simulink model "axi_qpsk_rx_dec"  (R2017b)
settings: Solver=VariableStepAuto  StartTime=0.0  StopTime=10.0  RelTol=1e-3
PreLoadFcn:
  | design_filters_rx;      % run script to generate filter designs.
  | 
  | Rb = 1000;   % 1kbit / s
  | 
  | Rsym = Rb/2;   % 2 bits per symbol
  | 
  | Rsymbol = Rb/2;
  | 
  | OSR = 32;
  | 
  | f_error = 120;
  | 
  | fc = 100e3;
InitFcn:
  | fs_in=25.6e6;
values from neighbouring files (symbols this model uses):
  R_CIC = 3200    [design_filters_rx.m]
  R_CICcomp = 2    [design_filters_rx.m]
  R_HB = 2    [design_filters_rx.m]
  R_RRC = 4    [design_filters_rx.m]
undefined symbols (not defined in the file or in its folder): AXI4, designMultirateFIR, Lite
libraries: xbsIndex_r4 x70, dspmlti4 x12, dsparch4 x2, dspsrcs4 x2, commrandsrc2 x1, commdigbbndpm3 x1
settings Model: SimulationMode=accelerator  Creator=jgoldsmi  LastModifiedBy=josh

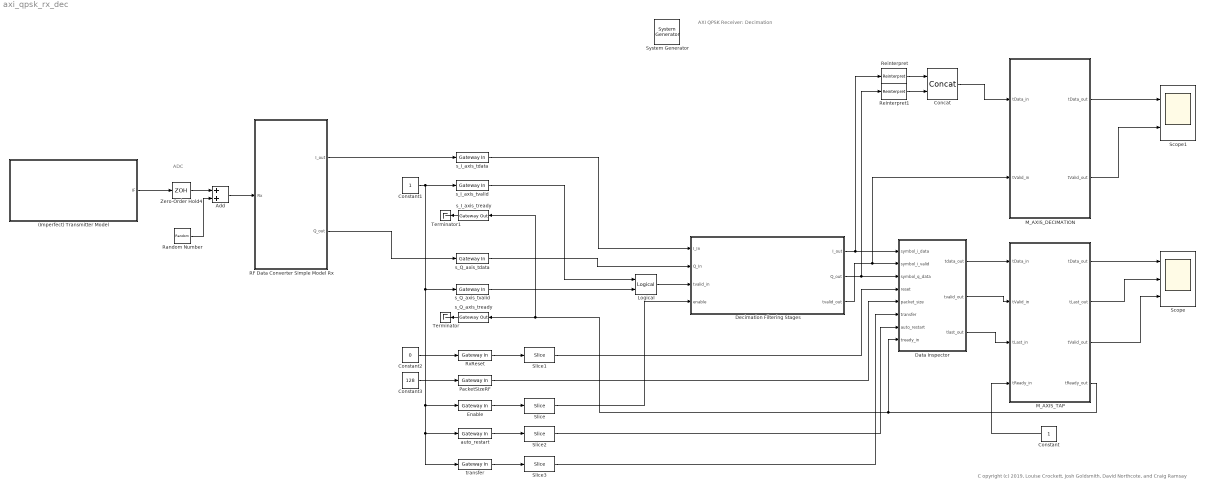
== system axi_qpsk_rx_dec ==
  note: ADC
  note: C opyright (c) 2019, Louise Crockett, Josh Goldsmith, David Northcote, and Craig Ramsay
  note: AXI QPSK Receiver:
      | Decimation
  " System Generator" : xbsIndex_r4/ System Generator  Tag=genX  xilinxfamily=zynquplusRFSOC  part=xczu28dr  speed=-2-e  package=ffvg1517  synthesis_tool=Vivado  clock_wrapper=Clock Enables  directory=../iprepo/zcu111/rx/rx_decimation  proj_type=Vivado  Synth_file=Vivado Synthesis Defaults  Impl_file=Vivado Implementation Defaults  testbench=off  simulink_period=1/fs_in  sysclk_period=(1/fs_in)/1e-9  dcm_input_clock_period=10  incr_netlist=off  trim_vbits=Everywhere in SubSystem  dbl_ovrd=According to Block Masks  core_generation=According to Block Masks  run_coregen=off  deprecated_control=off  eval_field=0  block_type=sysgen
  (Imperfect) Transmitter Model : Subsystem  mask(Model of a QPSK Transmitter with Timing and Frequency Offsets){T_error=5, F_error=f_error, fc=fc}
      mask prompts: T_error "Timing Error (ppm)"; F_error "Frequency Error (Hz)"; fc "IF Carrier Frequency (Hz)"
      mask help:
      | Enter the timing and frequency offsets that apply to the received signal.
      |
      | Both of these can be negative or positive values. Negative means that the timing / frequency of the transmitter is lower than expected.
      mask init:
      | T_Offset = 1+(T_error/1e6);
      | F_Offset = F_error;
  Add : Sum
  Concat : xbsIndex_r4/Concat  num_inputs=2  dbl_ovrd=off  block_type=concat
  Constant : Constant  OutDataTypeStr=boolean  SampleTime=1/fs_in
  Constant1 : Constant  OutDataTypeStr=boolean  SampleTime=-1
  Constant2 : Constant  Value=0  OutDataTypeStr=boolean  SampleTime=-1
  Constant3 : Constant  Value=128  OutDataTypeStr=uint32  SampleTime=-1
  Data Inspector : Subsystem
  Decimation Filtering Stages : Subsystem
  Enable : xbsIndex_r4/Gateway In  gui_display_data_type=Fixed-point  arith_type=Unsigned  n_bits=32  bin_pt=0  preci_type=Single  exp_width=8  frac_width=24  rows=1  columns=1  quantization="Round  (unbiased: +/- Inf)"  overflow=Saturate  period=1/fs_in  UseAsADC=off  ADCChannel='1'  interface=AXI4-Lite  automatic_assignment=off  address_offset=8  intf_name=''  intf_description=''  default_value=0  timing_constraint=None  locs_specified=off  LOCs={}  io_standard={}  inherit_from_input=off  hdl_port=on  dbl_ovrd=off  block_type=gatewayin
  Logical : xbsIndex_r4/Logical  logical_function=AND  inputs=2  en=off  latency=1  precision=Full  arith_type=Unsigned  n_bits=16  bin_pt=0  align_bp=on  dbl_ovrd=off  block_type=logical
  M_AXIS_DECIMATION : Subsystem
  M_AXIS_TAP : Subsystem
  PacketSizeRF : xbsIndex_r4/Gateway In  gui_display_data_type=Fixed-point  arith_type=Unsigned  n_bits=32  bin_pt=0  preci_type=Single  exp_width=8  frac_width=24  rows=1  columns=1  quantization=Truncate  overflow=Wrap  period=1/fs_in  UseAsADC=off  ADCChannel='1'  interface=AXI4-Lite  automatic_assignment=off  address_offset=4  intf_name=''  intf_description=''  default_value=0  timing_constraint=None  locs_specified=off  LOCs={}  io_standard={}  inherit_from_input=off  hdl_port=on  dbl_ovrd=off  block_type=gatewayin
  RF Data Converter Simple Model Rx : Subsystem
  Random Number : RandomNumber  Variance=0.05  SampleTime=1/(0.5*R_RRC*R_HB*R_CICcomp*R_CIC*8*Rb)
  Reinterpret : xbsIndex_r4/Reinterpret  force_arith_type=on  arith_type=Unsigned  force_bin_pt=on  bin_pt=0  block_type=reinterpret
  Reinterpret1 : xbsIndex_r4/Reinterpret  force_arith_type=on  arith_type=Unsigned  force_bin_pt=on  bin_pt=0  block_type=reinterpret
  RxReset : xbsIndex_r4/Gateway In  gui_display_data_type=Fixed-point  arith_type=Unsigned  n_bits=32  bin_pt=0  preci_type=Single  exp_width=8  frac_width=24  rows=1  columns=1  quantization="Round  (unbiased: +/- Inf)"  overflow=Saturate  period=1/fs_in  UseAsADC=off  ADCChannel='1'  interface=AXI4-Lite  automatic_assignment=off  address_offset=0  intf_name=''  intf_description=''  default_value=0  timing_constraint=None  locs_specified=off  LOCs={}  io_standard={}  inherit_from_input=off  hdl_port=on  dbl_ovrd=off  block_type=gatewayin
  Scope : Scope  NumInputPorts=3
  Scope1 : Scope  NumInputPorts=2
  Slice{,1..3} (4 alike) : xbsIndex_r4/Slice  nbits=1  boolean_output=on  mode=Two Bit Locations  bit1=0  base1=LSB of Input  bit0=0  base0=LSB of Input  dbl_ovrd=off  block_type=slice
  Terminator : Terminator
  Terminator1 : Terminator
  Zero-Order Hold4 : ZeroOrderHold  SampleTime=1/(0.5*R_RRC*R_HB*R_CICcomp*R_CIC*8*Rb)
  auto_restart : xbsIndex_r4/Gateway In  gui_display_data_type=Fixed-point  arith_type=Unsigned  n_bits=32  bin_pt=0  preci_type=Single  exp_width=8  frac_width=24  rows=1  columns=1  quantization="Round  (unbiased: +/- Inf)"  overflow=Saturate  period=1/fs_in  UseAsADC=off  ADCChannel='1'  interface=AXI4-Lite  automatic_assignment=off  address_offset=12  intf_name=''  intf_description=''  default_value=0  timing_constraint=None  locs_specified=off  LOCs={}  io_standard={}  inherit_from_input=off  hdl_port=on  dbl_ovrd=off  block_type=gatewayin
  s_I_axis_tdata : xbsIndex_r4/Gateway In  gui_display_data_type=Fixed-point  arith_type="Signed  (2's comp)"  n_bits=16  bin_pt=14  preci_type=Single  exp_width=8  frac_width=24  rows=1  columns=1  quantization="Round  (unbiased: +/- Inf)"  overflow=Saturate  period=1/fs_in  UseAsADC=off  ADCChannel='1'  interface=None  automatic_assignment=on  address_offset=hex2dec('00')  intf_name=''  intf_description=''  default_value=0  timing_constraint=None  locs_specified=off  LOCs={}  io_standard={}  inherit_from_input=off  hdl_port=on  dbl_ovrd=off  block_type=gatewayin
  s_I_axis_tready : xbsIndex_r4/Gateway Out  inherit_from_input=off  hdl_port=on  rows=1  columns=1  UseAsDAC=off  DACChannel='1'  interface=None  automatic_assignment=on  address_offset=hex2dec('00')  intf_name=''  intf_description=''  timing_constraint=None  locs_specified=off  LOCs={}  io_standard={}  block_type=gatewayout
  s_I_axis_tvalid : xbsIndex_r4/Gateway In  gui_display_data_type=Boolean  arith_type=Boolean  n_bits=32  bin_pt=0  preci_type=Single  exp_width=8  frac_width=24  rows=1  columns=1  quantization="Round  (unbiased: +/- Inf)"  overflow=Saturate  period=1/fs_in  UseAsADC=off  ADCChannel='1'  interface=None  automatic_assignment=on  address_offset=hex2dec('00')  intf_name=''  intf_description=''  default_value=0  timing_constraint=None  locs_specified=off  LOCs={}  io_standard={}  inherit_from_input=off  hdl_port=on  dbl_ovrd=off  block_type=gatewayin
  s_Q_axis_tdata : xbsIndex_r4/Gateway In  gui_display_data_type=Fixed-point  arith_type="Signed  (2's comp)"  n_bits=16  bin_pt=14  preci_type=Single  exp_width=8  frac_width=24  rows=1  columns=1  quantization="Round  (unbiased: +/- Inf)"  overflow=Saturate  period=1/fs_in  UseAsADC=off  ADCChannel='1'  interface=None  automatic_assignment=on  address_offset=hex2dec('00')  intf_name=''  intf_description=''  default_value=0  timing_constraint=None  locs_specified=off  LOCs={}  io_standard={}  inherit_from_input=off  hdl_port=on  dbl_ovrd=off  block_type=gatewayin
  s_Q_axis_tready : xbsIndex_r4/Gateway Out  inherit_from_input=off  hdl_port=on  rows=1  columns=1  UseAsDAC=off  DACChannel='1'  interface=None  automatic_assignment=on  address_offset=hex2dec('00')  intf_name=''  intf_description=''  timing_constraint=None  locs_specified=off  LOCs={}  io_standard={}  block_type=gatewayout
  s_Q_axis_tvalid : xbsIndex_r4/Gateway In  gui_display_data_type=Boolean  arith_type=Boolean  n_bits=32  bin_pt=0  preci_type=Single  exp_width=8  frac_width=24  rows=1  columns=1  quantization="Round  (unbiased: +/- Inf)"  overflow=Saturate  period=1/fs_in  UseAsADC=off  ADCChannel='1'  interface=None  automatic_assignment=on  address_offset=hex2dec('00')  intf_name=''  intf_description=''  default_value=0  timing_constraint=None  locs_specified=off  LOCs={}  io_standard={}  inherit_from_input=off  hdl_port=on  dbl_ovrd=off  block_type=gatewayin
  transfer : xbsIndex_r4/Gateway In  gui_display_data_type=Fixed-point  arith_type=Unsigned  n_bits=32  bin_pt=0  preci_type=Single  exp_width=8  frac_width=24  rows=1  columns=1  quantization="Round  (unbiased: +/- Inf)"  overflow=Saturate  period=1/fs_in  UseAsADC=off  ADCChannel='1'  interface=AXI4-Lite  automatic_assignment=off  address_offset=16  intf_name=''  intf_description=''  default_value=0  timing_constraint=None  locs_specified=off  LOCs={}  io_standard={}  inherit_from_input=off  hdl_port=on  dbl_ovrd=off  block_type=gatewayin
  wires:
  Decimation Filtering Stages/1(I_out) -> Data Inspector/1(symbol_i_data), Reinterpret/1
  Decimation Filtering Stages/2(Q_out) -> Reinterpret1/1, Data Inspector/3(symbol_q_data)
  Decimation Filtering Stages/3(tvalid_out) -> M_AXIS_DECIMATION/2(tValid_in), Data Inspector/2(symbol_i_valid)
  Zero-Order Hold4/1 -> Add/1
  (Imperfect) Transmitter Model/1(IF) -> Zero-Order Hold4/1
  Random Number/1 -> Add/2
  Add/1 -> RF Data Converter Simple Model Rx/1(Rx)
  RxReset/1 -> Slice1/1
  transfer/1 -> Slice3/1
  Enable/1 -> Slice/1
  auto_restart/1 -> Slice2/1
  s_I_axis_tdata/1 -> Decimation Filtering Stages/1(I_In)
  s_Q_axis_tdata/1 -> Decimation Filtering Stages/2(Q_In)
  s_I_axis_tvalid/1 -> Logical/1
  s_Q_axis_tvalid/1 -> Logical/2
  Logical/1 -> Decimation Filtering Stages/3(tvalid_in)
  Slice/1 -> Decimation Filtering Stages/4(enable)
  Slice2/1 -> Data Inspector/7(auto_restart)
  Slice3/1 -> Data Inspector/6(transfer)
  PacketSizeRF/1 -> Data Inspector/5(packet_size)
  Slice1/1 -> Data Inspector/4(reset)
  Data Inspector/1(tdata_out) -> M_AXIS_TAP/1(tData_in)
  Data Inspector/2(tvalid_out) -> M_AXIS_TAP/2(tValid_in)
  Data Inspector/3(tlast_out) -> M_AXIS_TAP/3(tLast_in)
  Constant/1 -> M_AXIS_TAP/4(tReady_in)
  M_AXIS_TAP/4(tReady_out) -> Data Inspector/8(tready_in), s_Q_axis_tready/1, s_I_axis_tready/1
  RF Data Converter Simple Model Rx/1(I_out) -> s_I_axis_tdata/1
  RF Data Converter Simple Model Rx/2(Q_out) -> s_Q_axis_tdata/1
  s_Q_axis_tready/1 -> Terminator/1
  s_I_axis_tready/1 -> Terminator1/1
  Constant1/1 -> s_I_axis_tvalid/1, transfer/1, auto_restart/1, Enable/1, s_Q_axis_tvalid/1
  Constant2/1 -> RxReset/1
  Constant3/1 -> PacketSizeRF/1
  M_AXIS_TAP/1(tData_out) -> Scope/1
  M_AXIS_TAP/2(tLast_out) -> Scope/2
  M_AXIS_TAP/3(tValid_out) -> Scope/3
  M_AXIS_DECIMATION/1(tData_out) -> Scope1/1
  M_AXIS_DECIMATION/2(tValid_out) -> Scope1/2
  Concat/1 -> M_AXIS_DECIMATION/1(tData_in)
  Reinterpret/1 -> Concat/1
  Reinterpret1/1 -> Concat/2

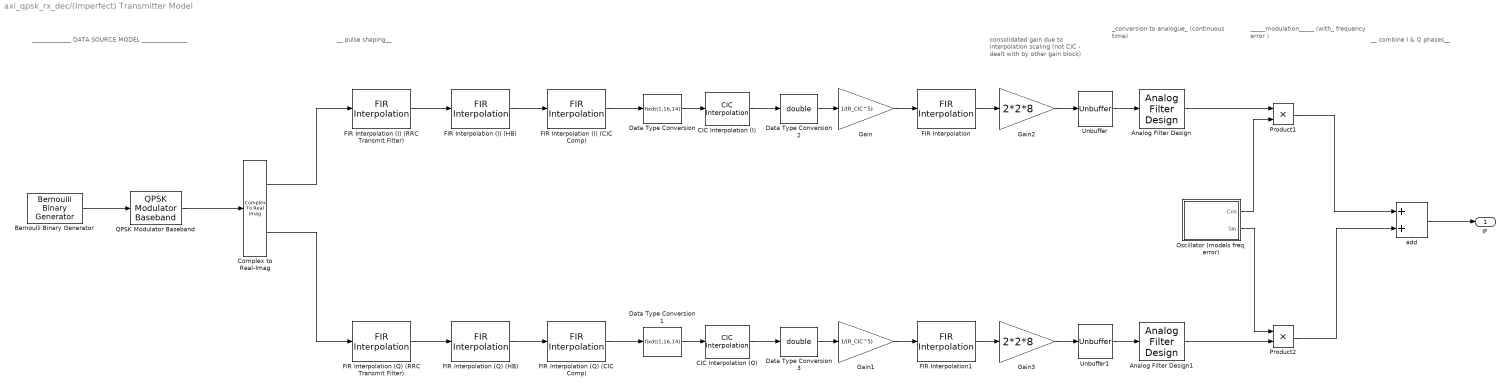
== system axi_qpsk_rx_dec/(Imperfect) Transmitter Model ==
  note: consolidated gain
      | due to interpolation scaling
      | (not CIC - dealt with by other
      | gain block)
  note: _____________ DATA SOURCE MODEL _______________
  note: _conversion to analogue_
      | (continuous time)
  note: __ pulse shaping__
  note: _____modulation_____
      | (with_ frequency error )
  note: __ combine I & Q phases__
  Analog Filter Design : dsparch4/Analog Filter Design  method=Butterworth  filttype=Lowpass  N=8  Wlo=2*pi*Rsymbol*T_Offset  Whi=80  Rp=2  Rs=40
  Analog Filter Design1 : dsparch4/Analog Filter Design  method=Butterworth  filttype=Lowpass  N=8  Wlo=2*pi*Rsymbol*T_Offset  Whi=80  Rp=2  Rs=40
  Bernoulli Binary Generator : commrandsrc2/Bernoulli Binary Generator  P=0.5  seed=61  Ts=1/(T_Offset*Rb)  frameBased=on  sampPerFrame=2  orient=off  outDataType=double
  CIC Interpolation (I) : dspmlti4/CIC Interpolation  filtFrom=Dialog  filtobj=CICINTERP  ftype=Interpolator  R=R_CIC  M=1  N=5  filterInternals=Full precision  BPS=[16 16 16 16]  FLPS=0  outputWordLength=32  outputFracLength=0  launchFVT=off  framing=Enforce single-rate processing  InputProcessing=Columns as channels (frame based)  OutputFrames=off
      settings: SourceProductName=DSP System Toolbox  SourceProductBaseCode=DS
  CIC Interpolation (Q) : dspmlti4/CIC Interpolation  filtFrom=Dialog  filtobj=CICINTERP  ftype=Interpolator  R=R_CIC  M=1  N=5  filterInternals=Full precision  BPS=[16 16 16 16]  FLPS=0  outputWordLength=32  outputFracLength=0  launchFVT=off  framing=Enforce single-rate processing  InputProcessing=Columns as channels (frame based)  OutputFrames=off
      settings: SourceProductName=DSP System Toolbox  SourceProductBaseCode=DS
  Complex to Real-Imag : ComplexToRealImag
  Data Type Conversion : DataTypeConversion  OutDataTypeStr=fixdt(1,16,14)
  Data Type Conversion1 : DataTypeConversion  OutDataTypeStr=fixdt(1,16,14)
  Data Type Conversion2 : DataTypeConversion  OutDataTypeStr=double
  Data Type Conversion3 : DataTypeConversion  OutDataTypeStr=double
  FIR Interpolation : dspmlti4/FIR Interpolation  FilterSource=Auto  h=designMultirateFIR(3,1)  L=8  FilterObject=FINTERP  InputProcessing=Columns as channels (frame based)  framing=Allow multirate processing  outputBufInitCond=0  roundingMode=Floor  overflowMode=off  firstCoeffDataTypeStr=Inherit: Same word length as input  firstCoeffMin=[]  firstCoeffMax=[]  firstCoeffLastDataTypeStr=Inherit: Same word length as input  outputDataTypeStr=Inherit: Same as accumulator  outputMin=[]  outputMax=[]  outputLastDataTypeStr=Inherit: Same as accumulator
      settings: SourceProductName=DSP System Toolbox
  FIR Interpolation1 : dspmlti4/FIR Interpolation  FilterSource=Auto  h=designMultirateFIR(3,1)  L=8  FilterObject=FINTERP  InputProcessing=Columns as channels (frame based)  framing=Allow multirate processing  outputBufInitCond=0  roundingMode=Floor  overflowMode=off  firstCoeffDataTypeStr=Inherit: Same word length as input  firstCoeffMin=[]  firstCoeffMax=[]  firstCoeffLastDataTypeStr=Inherit: Same word length as input  outputDataTypeStr=Inherit: Same as accumulator  outputMin=[]  outputMax=[]  outputLastDataTypeStr=Inherit: Same as accumulator
      settings: SourceProductName=DSP System Toolbox
  FIR Interpolation (I) (CIC Comp) : dspmlti4/FIR Interpolation  FilterSource=Dialog parameters  h=WComp.Numerator  L=R_CICcomp  FilterObject=FINTERP  InputProcessing=Columns as channels (frame based)  framing=Allow multirate processing  outputBufInitCond=0  roundingMode=Floor  overflowMode=off  firstCoeffDataTypeStr=Inherit: Same word length as input  firstCoeffMin=[]  firstCoeffMax=[]  firstCoeffLastDataTypeStr=Inherit: Same word length as input  outputDataTypeStr=Inherit: Same as accumulator  outputMin=[]  outputMax=[]  outputLastDataTypeStr=Inherit: Same as accumulator
      settings: SourceProductName=DSP System Toolbox
  FIR Interpolation (I) (HB) : dspmlti4/FIR Interpolation  FilterSource=Dialog parameters  h=HB.Numerator  L=2  FilterObject=FINTERP  InputProcessing=Columns as channels (frame based)  framing=Allow multirate processing  outputBufInitCond=0  roundingMode=Floor  overflowMode=off  firstCoeffDataTypeStr=Inherit: Same word length as input  firstCoeffMin=[]  firstCoeffMax=[]  firstCoeffLastDataTypeStr=Inherit: Same word length as input  outputDataTypeStr=Inherit: Same as accumulator  outputMin=[]  outputMax=[]  outputLastDataTypeStr=Inherit: Same as accumulator
      settings: SourceProductName=DSP System Toolbox
  FIR Interpolation (I) (RRC Transmit Filter) : dspmlti4/FIR Interpolation  FilterSource=Dialog parameters  h=WRRC.Numerator  L=R_RRC  FilterObject=FINTERP  InputProcessing=Columns as channels (frame based)  framing=Allow multirate processing  outputBufInitCond=0  roundingMode=Floor  overflowMode=off  firstCoeffDataTypeStr=Inherit: Same word length as input  firstCoeffMin=[]  firstCoeffMax=[]  firstCoeffLastDataTypeStr=Inherit: Same word length as input  outputDataTypeStr=Inherit: Same as accumulator  outputMin=[]  outputMax=[]  outputLastDataTypeStr=Inherit: Same as accumulator
      settings: SourceProductName=DSP System Toolbox
  FIR Interpolation (Q) (CIC Comp) : dspmlti4/FIR Interpolation  FilterSource=Dialog parameters  h=WComp.Numerator  L=R_CICcomp  FilterObject=FINTERP  InputProcessing=Columns as channels (frame based)  framing=Allow multirate processing  outputBufInitCond=0  roundingMode=Floor  overflowMode=off  firstCoeffDataTypeStr=Inherit: Same word length as input  firstCoeffMin=[]  firstCoeffMax=[]  firstCoeffLastDataTypeStr=Inherit: Same word length as input  outputDataTypeStr=Inherit: Same as accumulator  outputMin=[]  outputMax=[]  outputLastDataTypeStr=Inherit: Same as accumulator
      settings: SourceProductName=DSP System Toolbox
  FIR Interpolation (Q) (HB) : dspmlti4/FIR Interpolation  FilterSource=Dialog parameters  h=HB.Numerator  L=2  FilterObject=FINTERP  InputProcessing=Columns as channels (frame based)  framing=Allow multirate processing  outputBufInitCond=0  roundingMode=Floor  overflowMode=off  firstCoeffDataTypeStr=Inherit: Same word length as input  firstCoeffMin=[]  firstCoeffMax=[]  firstCoeffLastDataTypeStr=Inherit: Same word length as input  outputDataTypeStr=Inherit: Same as accumulator  outputMin=[]  outputMax=[]  outputLastDataTypeStr=Inherit: Same as accumulator
      settings: SourceProductName=DSP System Toolbox
  FIR Interpolation (Q) (RRC Transmit Filter) : dspmlti4/FIR Interpolation  FilterSource=Dialog parameters  h=WRRC.Numerator  L=R_RRC  FilterObject=FINTERP  InputProcessing=Columns as channels (frame based)  framing=Allow multirate processing  outputBufInitCond=0  roundingMode=Floor  overflowMode=off  firstCoeffDataTypeStr=Inherit: Same word length as input  firstCoeffMin=[]  firstCoeffMax=[]  firstCoeffLastDataTypeStr=Inherit: Same word length as input  outputDataTypeStr=Inherit: Same as accumulator  outputMin=[]  outputMax=[]  outputLastDataTypeStr=Inherit: Same as accumulator
      settings: SourceProductName=DSP System Toolbox
  Gain : Gain  Gain=1/(R_CIC^5)
  Gain1 : Gain  Gain=1/(R_CIC^5)
  Gain2 : Gain  Gain=2*2*8
  Gain3 : Gain  Gain=2*2*8
  Oscillator (models freq. error) : Subsystem
  Product1 : Product
  Product2 : Product
  QPSK Modulator Baseband : commdigbbndpm3/QPSK Modulator Baseband  InType=Bit  Enc=Gray  Ph=pi/4  outDtype=double  outWordLen=16  outUDDataType=sfix(16)  outFracLenMode=Best precision  outFracLen=15  outDataTypeStr=double  outLastDataTypeStr=double
  Unbuffer : Unbuffer
  Unbuffer1 : Unbuffer
  add : Sum
  IF : Outport
  wires:
  FIR Interpolation (Q) (RRC Transmit Filter)/1 -> FIR Interpolation (Q) (HB)/1
  Complex to Real-Imag/2 -> FIR Interpolation (Q) (RRC Transmit Filter)/1
  Complex to Real-Imag/1 -> FIR Interpolation (I) (RRC Transmit Filter)/1
  Bernoulli Binary Generator/1 -> QPSK Modulator Baseband/1
  FIR Interpolation (I) (RRC Transmit Filter)/1 -> FIR Interpolation (I) (HB)/1
  Product1/1 -> add/1
  Analog Filter Design/1 -> Product1/1
  Analog Filter Design1/1 -> Product2/2
  Product2/1 -> add/2
  add/1 -> IF/1
  Oscillator (models freq. error)/1(Cos) -> Product1/2
  Oscillator (models freq. error)/2(Sin) -> Product2/1
  QPSK Modulator Baseband/1 -> Complex to Real-Imag/1
  Unbuffer/1 -> Analog Filter Design/1
  Unbuffer1/1 -> Analog Filter Design1/1
  FIR Interpolation (I) (HB)/1 -> FIR Interpolation (I) (CIC Comp)/1
  FIR Interpolation (Q) (HB)/1 -> FIR Interpolation (Q) (CIC Comp)/1
  FIR Interpolation (I) (CIC Comp)/1 -> Data Type Conversion/1
  FIR Interpolation (Q) (CIC Comp)/1 -> Data Type Conversion1/1
  CIC Interpolation (I)/1 -> Data Type Conversion2/1
  CIC Interpolation (Q)/1 -> Data Type Conversion3/1
  FIR Interpolation/1 -> Gain2/1
  FIR Interpolation1/1 -> Gain3/1
  Data Type Conversion/1 -> CIC Interpolation (I)/1
  Data Type Conversion1/1 -> CIC Interpolation (Q)/1
  Data Type Conversion2/1 -> Gain/1
  Data Type Conversion3/1 -> Gain1/1
  Gain/1 -> FIR Interpolation/1
  Gain1/1 -> FIR Interpolation1/1
  Gain2/1 -> Unbuffer/1
  Gain3/1 -> Unbuffer1/1

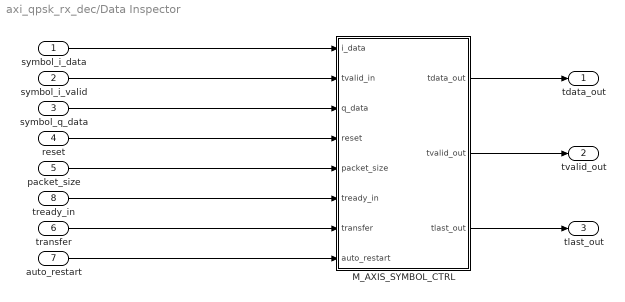
== system axi_qpsk_rx_dec/Data Inspector ==
  symbol_i_data : Inport
  symbol_i_valid : Inport  Port=2
  symbol_q_data : Inport  Port=3
  reset : Inport  Port=4
  packet_size : Inport  Port=5
  transfer : Inport  Port=6
  auto_restart : Inport  Port=7
  tready_in : Inport  Port=8
  M_AXIS_SYMBOL_CTRL : Subsystem
  tdata_out : Outport
  tvalid_out : Outport  Port=2
  tlast_out : Outport  Port=3
  wires:
  auto_restart/1 -> M_AXIS_SYMBOL_CTRL/8(auto_restart)
  transfer/1 -> M_AXIS_SYMBOL_CTRL/7(transfer)
  M_AXIS_SYMBOL_CTRL/3(tlast_out) -> tlast_out/1
  M_AXIS_SYMBOL_CTRL/2(tvalid_out) -> tvalid_out/1
  M_AXIS_SYMBOL_CTRL/1(tdata_out) -> tdata_out/1
  tready_in/1 -> M_AXIS_SYMBOL_CTRL/6(tready_in)
  packet_size/1 -> M_AXIS_SYMBOL_CTRL/5(packet_size)
  reset/1 -> M_AXIS_SYMBOL_CTRL/4(reset)
  symbol_q_data/1 -> M_AXIS_SYMBOL_CTRL/3(q_data)
  symbol_i_valid/1 -> M_AXIS_SYMBOL_CTRL/2(tvalid_in)
  symbol_i_data/1 -> M_AXIS_SYMBOL_CTRL/1(i_data)

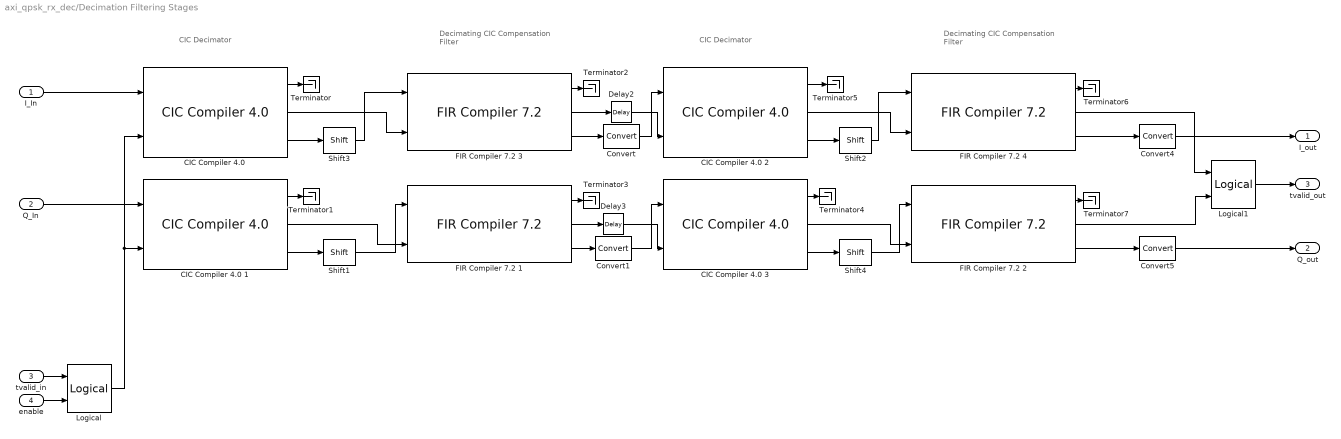
== system axi_qpsk_rx_dec/Decimation Filtering Stages ==
  note: CIC Decimator
  note: Decimating CIC
      | Compensation Filter
  note: CIC Decimator
  note: Decimating CIC
      | Compensation Filter
  I_In : Inport
  Q_In : Inport  Port=2
  tvalid_in : Inport  Port=3
  enable : Inport  Port=4
  "CIC Compiler 4.0 " : xbsIndex_r4/CIC Compiler 4.0   filter_type=Decimation  number_of_stages=3  differential_delay=1  number_of_channels=1  sample_rate_changes=Fixed  fixed_or_initial_rate=R_CIC_i  minimum_rate=40  maximum_rate=40  ratespecification=Maximum_Possible  sampleperiod=1  hardwareoversamplingrate=1  quantization=Full_Precision  output_data_width=34  use_xtreme_dsp_slice=on  use_streaming_interface=on  has_aclken=on  has_aresetn=off  has_dout_tready=off  trim_axipin_name=on  gui_behaviour=Sysgen_GUI  input_data_width=18  ip_name=CIC Compiler  ip_version=4.0  dsptool_ready=true  wrapper_available=true  port_translation_map={ 'aclken' => 'en', 'aresetn' => 'rst' }  ipcore_xco_need_fpga_part=true  ipcore_verbose=false  block_type=cic_compiler_v4_0
  CIC Compiler 4.0 1 : xbsIndex_r4/CIC Compiler 4.0   filter_type=Decimation  number_of_stages=3  differential_delay=1  number_of_channels=1  sample_rate_changes=Fixed  fixed_or_initial_rate=R_CIC_i  minimum_rate=20  maximum_rate=20  ratespecification=Maximum_Possible  sampleperiod=1  hardwareoversamplingrate=1  quantization=Full_Precision  output_data_width=31  use_xtreme_dsp_slice=on  use_streaming_interface=on  has_aclken=on  has_aresetn=off  has_dout_tready=off  trim_axipin_name=on  gui_behaviour=Sysgen_GUI  input_data_width=18  ip_name=CIC Compiler  ip_version=4.0  dsptool_ready=true  wrapper_available=true  port_translation_map={ 'aclken' => 'en', 'aresetn' => 'rst' }  ipcore_xco_need_fpga_part=true  ipcore_verbose=false  block_type=cic_compiler_v4_0
  CIC Compiler 4.0 2 : xbsIndex_r4/CIC Compiler 4.0   filter_type=Decimation  number_of_stages=3  differential_delay=1  number_of_channels=1  sample_rate_changes=Fixed  fixed_or_initial_rate=R_CIC_i  minimum_rate=20  maximum_rate=20  ratespecification=Maximum_Possible  sampleperiod=1  hardwareoversamplingrate=1  quantization=Full_Precision  output_data_width=31  use_xtreme_dsp_slice=on  use_streaming_interface=on  has_aclken=on  has_aresetn=off  has_dout_tready=off  trim_axipin_name=on  gui_behaviour=Sysgen_GUI  input_data_width=18  ip_name=CIC Compiler  ip_version=4.0  dsptool_ready=true  wrapper_available=true  port_translation_map={ 'aclken' => 'en', 'aresetn' => 'rst' }  ipcore_xco_need_fpga_part=true  ipcore_verbose=false  block_type=cic_compiler_v4_0
  CIC Compiler 4.0 3 : xbsIndex_r4/CIC Compiler 4.0   filter_type=Decimation  number_of_stages=3  differential_delay=1  number_of_channels=1  sample_rate_changes=Fixed  fixed_or_initial_rate=R_CIC_i  minimum_rate=20  maximum_rate=20  ratespecification=Maximum_Possible  sampleperiod=1  hardwareoversamplingrate=1  quantization=Full_Precision  output_data_width=31  use_xtreme_dsp_slice=on  use_streaming_interface=on  has_aclken=on  has_aresetn=off  has_dout_tready=off  trim_axipin_name=on  gui_behaviour=Sysgen_GUI  input_data_width=18  ip_name=CIC Compiler  ip_version=4.0  dsptool_ready=true  wrapper_available=true  port_translation_map={ 'aclken' => 'en', 'aresetn' => 'rst' }  ipcore_xco_need_fpga_part=true  ipcore_verbose=false  block_type=cic_compiler_v4_0
  Convert{,1,4..5} (4 alike) : xbsIndex_r4/Convert  gui_display_data_type=Fixed-point  arith_type="Signed  (2's comp)"  n_bits=16  bin_pt=14  float_type=Single  exp_bits=8  fraction_bits=24  quantization=Truncate  overflow=Wrap  en=off  latency=1  pipeline=off  dbl_ovrd=off  block_type=convert
  Delay2 : xbsIndex_r4/Delay  rst=off  infoeditControl=Selection of Reset will increase slice count due to use of real FFs and instead of SRLs  en=off  latency=1  reg_retiming=off  dbl_ovrd=off  block_type=delay
  Delay3 : xbsIndex_r4/Delay  rst=off  infoeditControl=Selection of Reset will increase slice count due to use of real FFs and instead of SRLs  en=off  latency=1  reg_retiming=off  dbl_ovrd=off  block_type=delay
  FIR Compiler 7.2 {1..4} (4 alike) : xbsIndex_r4/FIR Compiler 7.2   coefficientvector=WComp_i.Numerator  coefficient_sets=1  coefficient_reload=off  filter_type=Decimation  rate_change_type=Integer  interpolation_rate=1  decimation_rate=2  zero_pack_factor=1  channel_sequence=Basic  number_channels=1  pattern_list='P4-0,P4-1,P4-2,P4-3,P4-4'  number_paths=1  ratespecification=Maximum_Possible  sampleperiod=3200  hardwareoversamplingrate=1  coefficient_sign=Signed  quantization=Quantize_Only  coefficient_width=16  bestprecision=on  coefficient_fractional_bits=15  coefficient_structure=Inferred  output_rounding_mode=Full_Precision  output_width=33  filter_architecture=Systolic_Multiply_Accumulate  optimization_goal=Area  optimization_list='None'  data_buffer_type=Automatic  coefficient_buffer_type=Automatic  input_buffer_type=Automatic  output_buffer_type=Automatic  preference_for_other_storage=Automatic  multi_column_support=Automatic  columnconfig='10'  inter_column_pipe_length=4  data_has_tlast=Not_Required  m_data_has_tready=off  s_data_has_fifo=off  s_data_has_tuser=Not_Required  m_data_has_tuser=Not_Required  s_config_sync_mode=On_Vector  s_config_method=Single  num_reload_slots=1  has_aclken=on  has_aresetn=off  infoeditControl=ARESETn must be asserted for a minimum of 2 cycles  reset_data_vector=on  trim_axipin_name=on  simulation_type=hybrid_sim  simulation_model=sysgen:xfirv7_2_cmodel  data_path_portlist={ 's_axis_data_tdata', 'm_axis_data_tdata' }  passband_min=0.0  passband_max=0.5  stopband_min=0.5  stopband_max=1.0  filter_selection=1  gui_behaviour='Sysgen_GUI'  data_sign=Signed  data_width=16  data_fractional_bits=0  data_tuser_width=1  wrapper_available=true  ip_wrap_arbitrary_binary_point=true  ip_name=FIR Compiler  ip_version=7.2  dsptool_ready=true  ipcore_usecache=true  ipcore_useipmodelcache=true  port_translation_map={ 'aclken' => 'en', 'aresetn' => 'rst' }  run_core_at_system_period=true  ipcore_xco_need_fpga_part=true  block_type=fir_compiler_v7_2
      settings: infoedit=Maximum Possible : Maximizes oversampling rate. Abstracted input handshake (no s_data_tvalid) and automatic rate propagation.<br>Hardware Oversampling Rate : Specifies oversampling rate relative to the input sample period. Abstracted input handshake (no s_data_tvalid) and automatic rate propagation.<br>Input/Output Sample Period : Specifies absolute oversampling rate. No input handshake abstraction (exposes s_data_tvalid) and no rate propagation.
  Logical : xbsIndex_r4/Logical  logical_function=AND  inputs=2  en=off  latency=0  precision=Full  arith_type=Unsigned  n_bits=16  bin_pt=0  align_bp=on  dbl_ovrd=off  block_type=logical
  Logical1 : xbsIndex_r4/Logical  logical_function=AND  inputs=2  en=off  latency=1  precision=Full  arith_type=Unsigned  n_bits=16  bin_pt=0  align_bp=on  dbl_ovrd=off  block_type=logical
  Shift{1..4} (4 alike) : xbsIndex_r4/Shift  shift_dir=Right  shift_bits=13  en=off  latency=0  precision=User Defined  arith_type="Signed  (2's comp)"  n_bits=16  bin_pt=14  quantization=Truncate  overflow=Wrap  dbl_ovrd=off  block_type=shift
  Terminator{,1..7} (8 alike) : Terminator
  I_out : Outport
  Q_out : Outport  Port=2
  tvalid_out : Outport  Port=3
  wires:
  FIR Compiler 7.2 1/3 -> Convert1/1
  CIC Compiler 4.0 1/3 -> Shift1/1
  "CIC Compiler 4.0 "/3 -> Shift3/1
  FIR Compiler 7.2 3/3 -> Convert/1
  Shift3/1 -> FIR Compiler 7.2 3/1
  Shift1/1 -> FIR Compiler 7.2 1/1
  Shift4/1 -> FIR Compiler 7.2 2/1
  Shift2/1 -> FIR Compiler 7.2 4/1
  CIC Compiler 4.0 2/3 -> Shift2/1
  CIC Compiler 4.0 3/3 -> Shift4/1
  Convert/1 -> CIC Compiler 4.0 2/1
  Convert1/1 -> CIC Compiler 4.0 3/1
  FIR Compiler 7.2 2/3 -> Convert5/1
  FIR Compiler 7.2 4/3 -> Convert4/1
  tvalid_in/1 -> Logical/1
  Logical/1 -> CIC Compiler 4.0 1/2, "CIC Compiler 4.0 "/2
  CIC Compiler 4.0 1/2 -> FIR Compiler 7.2 1/2
  "CIC Compiler 4.0 "/2 -> FIR Compiler 7.2 3/2
  FIR Compiler 7.2 3/2 -> Delay2/1
  Delay2/1 -> CIC Compiler 4.0 2/2
  FIR Compiler 7.2 1/2 -> Delay3/1
  Delay3/1 -> CIC Compiler 4.0 3/2
  CIC Compiler 4.0 2/2 -> FIR Compiler 7.2 4/2
  CIC Compiler 4.0 3/2 -> FIR Compiler 7.2 2/2
  Logical1/1 -> tvalid_out/1
  "CIC Compiler 4.0 "/1 -> Terminator/1
  CIC Compiler 4.0 1/1 -> Terminator1/1
  FIR Compiler 7.2 3/1 -> Terminator2/1
  FIR Compiler 7.2 1/1 -> Terminator3/1
  CIC Compiler 4.0 3/1 -> Terminator4/1
  CIC Compiler 4.0 2/1 -> Terminator5/1
  FIR Compiler 7.2 4/1 -> Terminator6/1
  FIR Compiler 7.2 2/1 -> Terminator7/1
  I_In/1 -> "CIC Compiler 4.0 "/1
  Q_In/1 -> CIC Compiler 4.0 1/1
  enable/1 -> Logical/2
  Convert4/1 -> I_out/1
  Convert5/1 -> Q_out/1
  FIR Compiler 7.2 4/2 -> Logical1/1
  FIR Compiler 7.2 2/2 -> Logical1/2

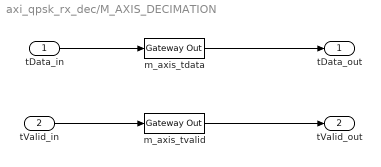
== system axi_qpsk_rx_dec/M_AXIS_DECIMATION ==
  tData_in : Inport
  tValid_in : Inport  Port=2
  m_axis_tdata : xbsIndex_r4/Gateway Out  inherit_from_input=off  hdl_port=on  rows=1  columns=1  UseAsDAC=off  DACChannel='1'  interface=None  automatic_assignment=on  address_offset=hex2dec('00')  intf_name=''  intf_description=''  timing_constraint=None  locs_specified=off  LOCs={}  io_standard={}  block_type=gatewayout
  m_axis_tvalid : xbsIndex_r4/Gateway Out  inherit_from_input=off  hdl_port=on  rows=1  columns=1  UseAsDAC=off  DACChannel='1'  interface=None  automatic_assignment=on  address_offset=hex2dec('00')  intf_name=''  intf_description=''  timing_constraint=None  locs_specified=off  LOCs={}  io_standard={}  block_type=gatewayout
  tData_out : Outport
  tValid_out : Outport  Port=2
  wires:
  m_axis_tvalid/1 -> tValid_out/1
  m_axis_tdata/1 -> tData_out/1
  tData_in/1 -> m_axis_tdata/1
  tValid_in/1 -> m_axis_tvalid/1

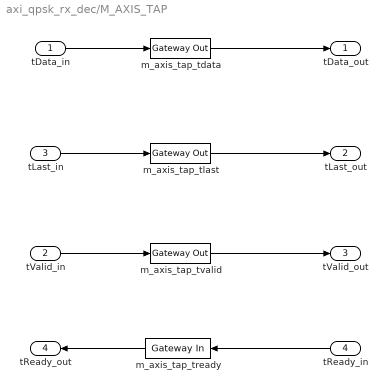
== system axi_qpsk_rx_dec/M_AXIS_TAP ==
  tData_in : Inport
  tValid_in : Inport  Port=2
  tLast_in : Inport  Port=3
  tReady_in : Inport  Port=4
  m_axis_tap_tdata : xbsIndex_r4/Gateway Out  inherit_from_input=off  hdl_port=on  rows=1  columns=1  UseAsDAC=off  DACChannel='1'  interface=None  automatic_assignment=on  address_offset=hex2dec('00')  intf_name=''  intf_description=''  timing_constraint=None  locs_specified=off  LOCs={}  io_standard={}  block_type=gatewayout
  m_axis_tap_tlast : xbsIndex_r4/Gateway Out  inherit_from_input=off  hdl_port=on  rows=1  columns=1  UseAsDAC=off  DACChannel='1'  interface=None  automatic_assignment=on  address_offset=hex2dec('00')  intf_name=''  intf_description=''  timing_constraint=None  locs_specified=off  LOCs={}  io_standard={}  block_type=gatewayout
  m_axis_tap_tready : xbsIndex_r4/Gateway In  gui_display_data_type=Boolean  arith_type=Boolean  n_bits=16  bin_pt=14  preci_type=Single  exp_width=8  frac_width=24  rows=1  columns=1  quantization="Round  (unbiased: +/- Inf)"  overflow=Saturate  period=1/fs_in  UseAsADC=off  ADCChannel='1'  interface=None  automatic_assignment=on  address_offset=hex2dec('00')  intf_name=''  intf_description=''  default_value=0  timing_constraint=None  locs_specified=off  LOCs={}  io_standard={}  inherit_from_input=off  hdl_port=on  dbl_ovrd=off  block_type=gatewayin
  m_axis_tap_tvalid : xbsIndex_r4/Gateway Out  inherit_from_input=off  hdl_port=on  rows=1  columns=1  UseAsDAC=off  DACChannel='1'  interface=None  automatic_assignment=on  address_offset=hex2dec('00')  intf_name=''  intf_description=''  timing_constraint=None  locs_specified=off  LOCs={}  io_standard={}  block_type=gatewayout
  tData_out : Outport
  tLast_out : Outport  Port=2
  tValid_out : Outport  Port=3
  tReady_out : Outport  Port=4
  wires:
  m_axis_tap_tready/1 -> tReady_out/1
  tValid_in/1 -> m_axis_tap_tvalid/1
  tLast_in/1 -> m_axis_tap_tlast/1
  tData_in/1 -> m_axis_tap_tdata/1
  m_axis_tap_tdata/1 -> tData_out/1
  m_axis_tap_tvalid/1 -> tValid_out/1
  m_axis_tap_tlast/1 -> tLast_out/1
  tReady_in/1 -> m_axis_tap_tready/1

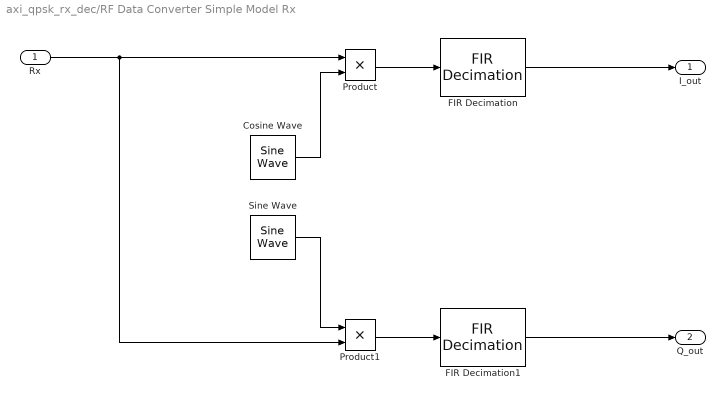
== system axi_qpsk_rx_dec/RF Data Converter Simple Model Rx ==
  Rx : Inport
  Cosine Wave : dspsrcs4/Sine Wave  Amplitude=1  Frequency=fc  Phase=pi/2  SampleMode=Discrete  OutComplex=Real  CompMethod=Trigonometric fcn  TableSize=Speed  SampleTime=1/(0.5*R_RRC*R_HB*R_CICcomp*R_CIC*8*Rb)  SamplesPerFrame=1  ResetState=Restart at time zero  OutputFrames=off  dataType=double  wordLen=16  udDataType=sfix(16)  fracBitsMode=Best precision  numFracBits=15  OutDataTypeStr=double  LastOutDataTypeStr=double
  FIR Decimation : dspmlti4/FIR Decimation  FilterSource=Auto  h=designMultirateFIR(1,2)  D=8  filtStruct=Direct form  FilterObject=FDECIM  framing=Enforce single-rate processing  inputOffset=0  outputBufInitCond=0  roundingMode=Floor  overflowMode=off  firstCoeffDataTypeStr=Inherit: Same word length as input  firstCoeffMin=[]  firstCoeffMax=[]  firstCoeffLastDataTypeStr=Inherit: Same word length as input  outputDataTypeStr=Inherit: Same as accumulator  outputMin=[]  outputMax=[]  outputLastDataTypeStr=Inherit: Same as accumulator
  FIR Decimation1 : dspmlti4/FIR Decimation  FilterSource=Auto  h=designMultirateFIR(1,2)  D=8  filtStruct=Direct form  FilterObject=FDECIM  framing=Enforce single-rate processing  inputOffset=0  outputBufInitCond=0  roundingMode=Floor  overflowMode=off  firstCoeffDataTypeStr=Inherit: Same word length as input  firstCoeffMin=[]  firstCoeffMax=[]  firstCoeffLastDataTypeStr=Inherit: Same word length as input  outputDataTypeStr=Inherit: Same as accumulator  outputMin=[]  outputMax=[]  outputLastDataTypeStr=Inherit: Same as accumulator
  Product : Product
  Product1 : Product
  Sine Wave : dspsrcs4/Sine Wave  Amplitude=1  Frequency=fc  Phase=pi  SampleMode=Discrete  OutComplex=Real  CompMethod=Trigonometric fcn  TableSize=Speed  SampleTime=1/(0.5*R_RRC*R_HB*R_CICcomp*R_CIC*8*Rb)  SamplesPerFrame=1  ResetState=Restart at time zero  OutputFrames=off  dataType=double  wordLen=16  udDataType=sfix(16)  fracBitsMode=Best precision  numFracBits=15  OutDataTypeStr=double  LastOutDataTypeStr=double
  I_out : Outport
  Q_out : Outport  Port=2
  wires:
  FIR Decimation/1 -> I_out/1
  Rx/1 -> Product1/2, Product/1
  Cosine Wave/1 -> Product/2
  Product/1 -> FIR Decimation/1
  Sine Wave/1 -> Product1/1
  Product1/1 -> FIR Decimation1/1
  FIR Decimation1/1 -> Q_out/1

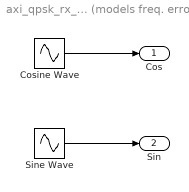
== system axi_qpsk_rx_dec/(Imperfect) Transmitter Model/Oscillator (models freq. error) ==
  Cosine Wave : Sin  Frequency=2*pi*(fc-F_Offset)  Phase=pi/2  SampleTime=0
  Sine Wave : Sin  Frequency=2*pi*(fc-F_Offset)  SampleTime=0
  Cos : Outport
  Sin : Outport  Port=2
  wires:
  Sine Wave/1 -> Sin/1
  Cosine Wave/1 -> Cos/1

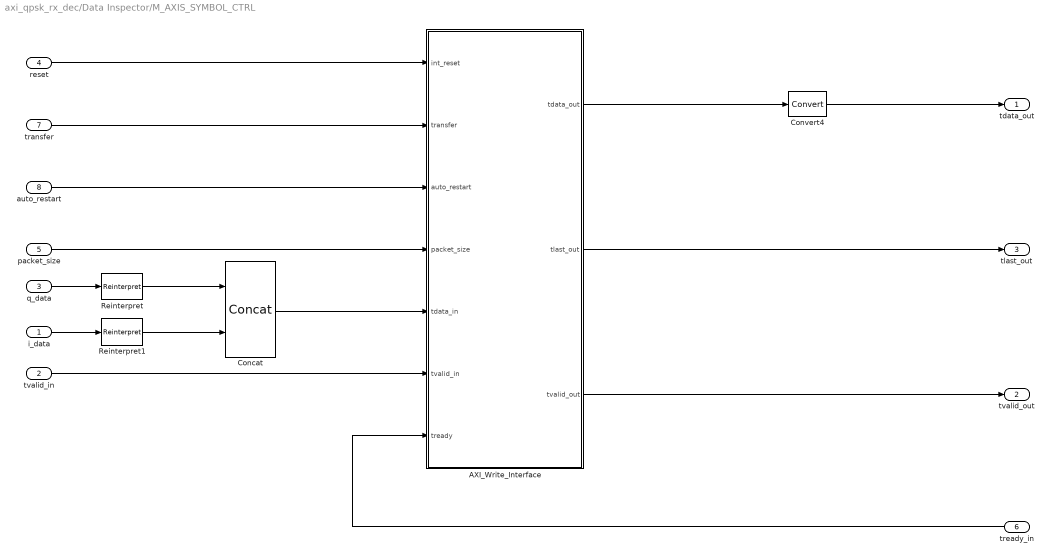
== system axi_qpsk_rx_dec/Data Inspector/M_AXIS_SYMBOL_CTRL ==
  i_data : Inport
  tvalid_in : Inport  Port=2
  q_data : Inport  Port=3
  reset : Inport  Port=4
  packet_size : Inport  Port=5
  tready_in : Inport  Port=6
  transfer : Inport  Port=7
  auto_restart : Inport  Port=8
  AXI_Write_Interface : Subsystem
  Concat : xbsIndex_r4/Concat  num_inputs=2  dbl_ovrd=off  block_type=concat
  Convert4 : xbsIndex_r4/Convert  gui_display_data_type=Fixed-point  arith_type=Unsigned  n_bits=32  bin_pt=0  float_type=Single  exp_bits=8  fraction_bits=24  quantization=Truncate  overflow=Wrap  en=off  latency=0  pipeline=off  dbl_ovrd=off  block_type=convert
  Reinterpret : xbsIndex_r4/Reinterpret  force_arith_type=on  arith_type=Unsigned  force_bin_pt=on  bin_pt=0  block_type=reinterpret
  Reinterpret1 : xbsIndex_r4/Reinterpret  force_arith_type=on  arith_type=Unsigned  force_bin_pt=on  bin_pt=0  block_type=reinterpret
  tdata_out : Outport
  tvalid_out : Outport  Port=2
  tlast_out : Outport  Port=3
  wires:
  Convert4/1 -> tdata_out/1
  AXI_Write_Interface/1(tdata_out) -> Convert4/1
  AXI_Write_Interface/3(tvalid_out) -> tvalid_out/1
  AXI_Write_Interface/2(tlast_out) -> tlast_out/1
  tready_in/1 -> AXI_Write_Interface/7(tready)
  auto_restart/1 -> AXI_Write_Interface/3(auto_restart)
  transfer/1 -> AXI_Write_Interface/2(transfer)
  Concat/1 -> AXI_Write_Interface/5(tdata_in)
  reset/1 -> AXI_Write_Interface/1(int_reset)
  tvalid_in/1 -> AXI_Write_Interface/6(tvalid_in)
  packet_size/1 -> AXI_Write_Interface/4(packet_size)
  Reinterpret/1 -> Concat/1
  Reinterpret1/1 -> Concat/2
  i_data/1 -> Reinterpret1/1
  q_data/1 -> Reinterpret/1

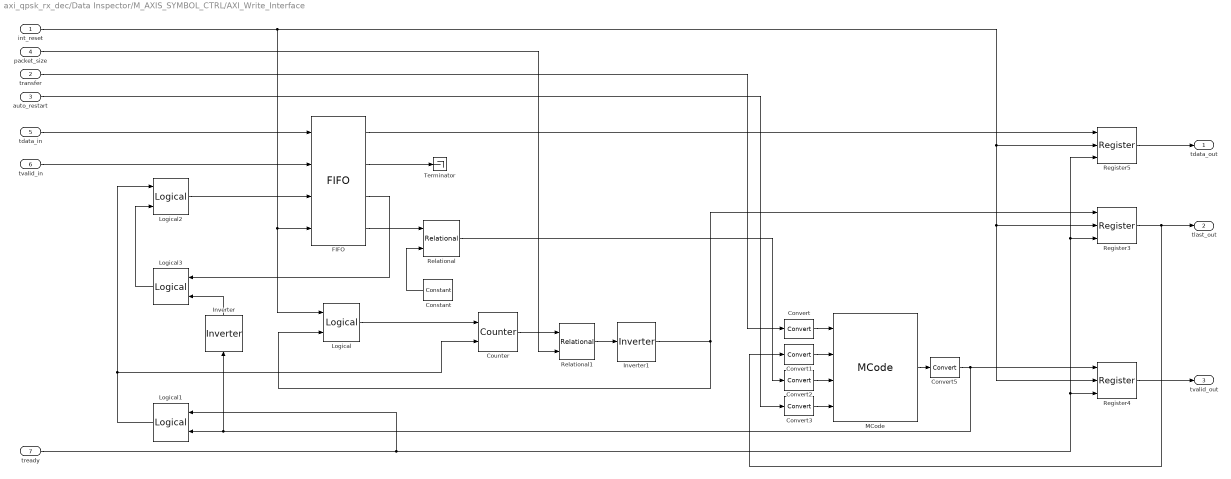
== system axi_qpsk_rx_dec/Data Inspector/M_AXIS_SYMBOL_CTRL/AXI_Write_Interface ==
  int_reset : Inport
  transfer : Inport  Port=2
  auto_restart : Inport  Port=3
  packet_size : Inport  Port=4
  tdata_in : Inport  Port=5
  tvalid_in : Inport  Port=6
  tready : Inport  Port=7
  Constant : xbsIndex_r4/Constant  const=256  gui_display_data_type=Fixed-point  arith_type=Unsigned  n_bits=11  bin_pt=0  preci_type=Single  exp_width=8  frac_width=24  explicit_period=on  period=1/fs_in  equ=P=C  opselect=C  inp2=PCIN>>17  opr=+  inp1=P  carry=CIN  dbl_ovrd=off  block_type=constant
  Convert{,1..3} (4 alike) : xbsIndex_r4/Convert  gui_display_data_type=Fixed-point  arith_type=Unsigned  n_bits=1  bin_pt=0  float_type=Single  exp_bits=8  fraction_bits=24  quantization=Truncate  overflow=Wrap  en=off  latency=0  pipeline=off  dbl_ovrd=off  block_type=convert
  Convert5 : xbsIndex_r4/Convert  gui_display_data_type=Boolean  arith_type=Boolean  n_bits=1  bin_pt=0  float_type=Single  exp_bits=8  fraction_bits=24  quantization=Truncate  overflow=Wrap  en=off  latency=0  pipeline=off  dbl_ovrd=off  block_type=convert
  Counter : xbsIndex_r4/Counter  cnt_type=Free Running  cnt_to=Inf  operation=Up  start_count=0  cnt_by_val=1  arith_type=Unsigned  n_bits=32  bin_pt=0  load_pin=off  rst=on  en=on  explicit_period=on  period=1/fs_in  use_behavioral_HDL=off  implementation=Fabric  dbl_ovrd=off  block_type=counter
  FIFO : xbsIndex_r4/FIFO  mem_type=Block RAM  performance_options=Standard_FIFO  embedded_registers=off  depth=512  percent_nbits=1  rst=on  rst_latency=2  en=off  use_dcount=on  use_percent_full_port=off  use_almost_empty=off  almost_empty_thresh=2  use_almost_full=off  almost_full_thresh=14  explicit_period=off  dbl_ovrd=off  block_type=fifo
  Inverter : xbsIndex_r4/Inverter  en=off  latency=0  dbl_ovrd=off  block_type=inv
  Inverter1 : xbsIndex_r4/Inverter  en=off  latency=0  dbl_ovrd=off  block_type=inv
  Logical : xbsIndex_r4/Logical  logical_function=OR  inputs=2  en=off  latency=0  precision=Full  arith_type=Unsigned  n_bits=16  bin_pt=0  align_bp=on  dbl_ovrd=off  block_type=logical
  Logical1 : xbsIndex_r4/Logical  logical_function=AND  inputs=2  en=off  latency=0  precision=Full  arith_type=Unsigned  n_bits=16  bin_pt=0  align_bp=on  dbl_ovrd=off  block_type=logical
  Logical2 : xbsIndex_r4/Logical  logical_function=OR  inputs=2  en=off  latency=0  precision=Full  arith_type=Unsigned  n_bits=16  bin_pt=0  align_bp=on  dbl_ovrd=off  block_type=logical
  Logical3 : xbsIndex_r4/Logical  logical_function=AND  inputs=2  en=off  latency=0  precision=Full  arith_type=Unsigned  n_bits=16  bin_pt=0  align_bp=on  dbl_ovrd=off  block_type=logical
  MCode : xbsIndex_r4/MCode  mfname=CtrlFSM  explicit_period=on  period=1/fs_in  inputsTable={'boundInpExpr'=>['','','',''],'inputs'=>['AXIwrite','tlast','dcount','AXIauto']}  outputsTable={'outputs'=>['re'],'suppressOut'=>['off']}  enable_stdout=off  enable_debug=off  suppress_output=on  defparams={}  hide_port_list={}  dbl_ovrd=off  block_type=mcode
  Register3 : xbsIndex_r4/Register  init=0  rst=on  en=on  dbl_ovrd=off  block_type=register
  Register4 : xbsIndex_r4/Register  init=0  rst=on  en=on  dbl_ovrd=off  block_type=register
  Register5 : xbsIndex_r4/Register  init=0  rst=on  en=on  dbl_ovrd=off  block_type=register
  Relational : xbsIndex_r4/Relational  mode=a>=b  op_type=Bool  en=off  latency=0  dbl_ovrd=off  block_type=relational
  Relational1 : xbsIndex_r4/Relational  mode=a<b  op_type=Bool  en=off  latency=0  dbl_ovrd=off  block_type=relational
  Terminator : Terminator
  tdata_out : Outport
  tlast_out : Outport  Port=2
  tvalid_out : Outport  Port=3
  wires:
  Register5/1 -> tdata_out/1
  FIFO/2 -> Terminator/1
  Logical2/1 -> FIFO/3
  Convert1/1 -> MCode/2
  Convert/1 -> MCode/1
  transfer/1 -> Convert/1
  int_reset/1 -> Logical/1, FIFO/4, Register5/2, Register3/2, Register4/2
  Inverter/1 -> Logical3/2
  tready/1 -> Register3/3, Register5/3, Register4/3, Logical1/1
  Convert3/1 -> MCode/4
  Convert2/1 -> MCode/3
  Inverter1/1 -> Logical/2, Register3/1
  Logical1/1 -> Logical2/1, Counter/2
  tdata_in/1 -> FIFO/1
  FIFO/3 -> Logical3/1
  Relational1/1 -> Inverter1/1
  Counter/1 -> Relational1/1
  Logical/1 -> Counter/1
  Relational/1 -> Convert2/1
  Constant/1 -> Relational/2
  packet_size/1 -> Relational1/2
  MCode/1 -> Convert5/1
  Logical3/1 -> Logical2/2
  auto_restart/1 -> Convert3/1
  FIFO/4 -> Relational/1
  Register3/1 -> Convert1/1, tlast_out/1
  Register4/1 -> tvalid_out/1
  Convert5/1 -> Register4/1, Inverter/1, Logical1/2
  FIFO/1 -> Register5/1
  tvalid_in/1 -> FIFO/2
